simulink model "DC_motor_comparison_28_01"  (R2019a)
settings: Solver=VariableStepAuto  StartTime=0.0  StopTime=50  RelTol=1e-3
undefined symbols (not defined in the file or in its folder): sigbuilder_block
libraries: simulink x4
settings Model: Creator=hp  LastModifiedBy=hp
settings SolverCC: AlgebraicLoopSolver=LineSearch

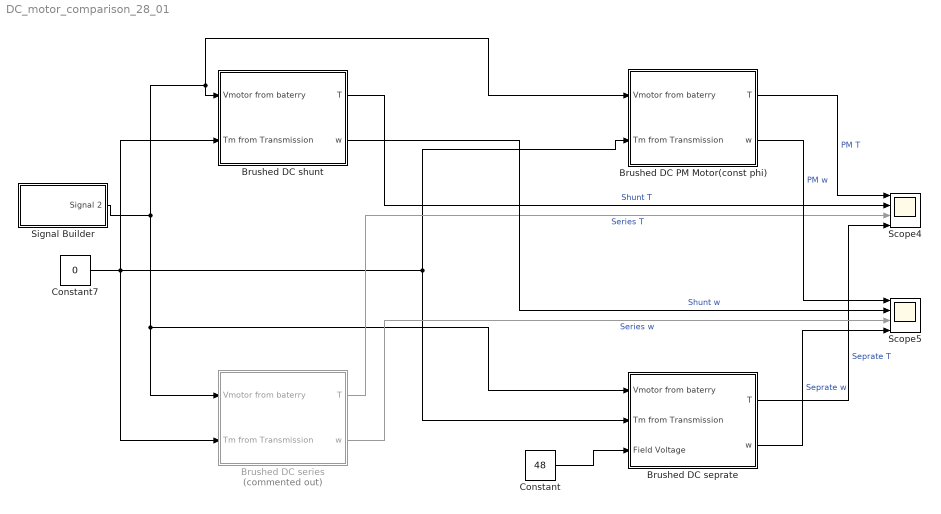
== system DC_motor_comparison_28_01 ==
  Brushed DC PM Motor(const phi) : Subsystem
  Brushed DC seprate : Subsystem
  Brushed DC series : Subsystem  Commented=on
  Brushed DC shunt : Subsystem
  Constant : Constant  Value=48
  Constant7 : Constant  Value=0
  Scope4 : Scope  NumInputPorts=4
  Scope5 : Scope  NumInputPorts=4
  Signal Builder : Subsystem  Tag=STV Subsys  LoadFcn=sigbuilder_block('load',[123.75 80.25 550.5 359.25 ]);  StartFcn=sigbuilder_block('start');  StopFcn=sigbuilder_block('stop');  ClipboardFcn=sigbuilder_block('clipboard');  mask(Sigbuilder block){tuvar=[0:10]}
      mask help: Simulink:masks:SigbuilderBlock_MD
      mask init:
      | if ~strcmp(get_param(bdroot(gcbh),'SimulationStatus'),'stopped') tuvar = sigbuilder_block('maskInit'); end
      settings: CopyFcn=sigbuilder_block('copy');  DeleteFcn=sigbuilder_block('delete');  ModelCloseFcn=sigbuilder_block('modelClose');  PreSaveFcn=sigbuilder_block('preSave');  PauseFcn=sigbuilder_block('pause');  ContinueFcn=sigbuilder_block('continue');  NameChangeFcn=sigbuilder_block('namechange');  OpenFcn=sigbuilder_block('open',[123.75 80.25 550.5 359.25 ]);  CloseFcn=sigbuilder_block('close');
      mask Display: plot(0, 0, 100, 100,[2, 2, 32, 32, 2], [68, 8, 8, 68, 68],[32, 2], [38, 38], [32, 19, 2],[53, 60, 44], [32, 17, 17, 2],[16, 16, 31, 31]);txt = getActiveGroup(gcbh);text(2, 100, txt,'verticalAlignment', 'top');
  wires:
  Signal Builder/1(Signal 2) -> Brushed DC series/1(Vmotor from baterry), Brushed DC seprate/1(Vmotor from baterry), Brushed DC PM Motor(const phi)/1(Vmotor from baterry), Brushed DC shunt/1(Vmotor from baterry)
  Constant7/1 -> Brushed DC series/2(Tm from Transmission), Brushed DC shunt/2(Tm from Transmission), Brushed DC seprate/2(Tm from Transmission), Brushed DC PM Motor(const phi)/2(Tm from Transmission)
  Brushed DC PM Motor(const phi)/1(T) -> Scope4/1  "PM T"
  Brushed DC shunt/1(T) -> Scope4/2  "Shunt T"
  Brushed DC series/1(T) -> Scope4/3  "Series T"
  Brushed DC seprate/1(T) -> Scope4/4  "Seprate T"
  Brushed DC seprate/2(w) -> Scope5/4  "Seprate w"
  Brushed DC series/2(w) -> Scope5/3  "Series w"
  Brushed DC PM Motor(const phi)/2(w) -> Scope5/1  "PM w"
  Brushed DC shunt/2(w) -> Scope5/2  "Shunt w"
  Constant/1 -> Brushed DC seprate/3(Field Voltage)

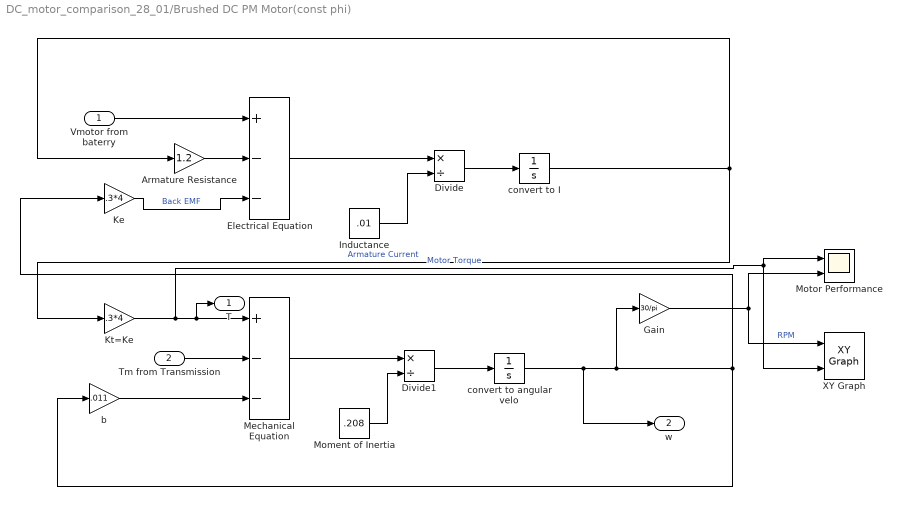
== system DC_motor_comparison_28_01/Brushed DC PM Motor(const phi) ==
  Vmotor from baterry : Inport
  Tm from Transmission : Inport  Port=2
  Armature Resistance : Gain  Gain=1.2
  Divide : Product  Inputs=*/
  Divide1 : Product  Inputs=*/
  Electrical Equation : Sum  Inputs=+--
  Gain : Gain  Gain=30/pi
  Inductance : Constant  Value=.01
  Ke : Gain  Gain=.3*4
  Kt=Ke : Gain  Gain=.3*4
  Mechanical Equation : Sum  Inputs=+--
  Moment of Inertia : Constant  Value=.208
  Motor Performance : Scope  NumInputPorts=2
  XY Graph : simulink/Sinks/XY Graph  xmin=0  xmax=12000  ymin=0  ymax=265  st=-1
  b : Gain  Gain=.011
  convert to angular velo : Integrator
  "convert to I " : Integrator
  T : Outport
  w : Outport  Port=2
  wires:
  Ke/1 -> Electrical Equation/3  "Back EMF"
  Divide/1 -> "convert to I "/1
  Armature Resistance/1 -> Electrical Equation/2
  Electrical Equation/1 -> Divide/1
  Inductance/1 -> Divide/2
  Mechanical Equation/1 -> Divide1/1
  "convert to I "/1 -> Armature Resistance/1, Kt=Ke/1  "Armature Current"
  Kt=Ke/1 -> XY Graph/2, Motor Performance/1, T/1, Mechanical Equation/1  "Motor Torque"
  convert to angular velo/1 -> Ke/1, b/1, Gain/1, w/1
  b/1 -> Mechanical Equation/3
  Moment of Inertia/1 -> Divide1/2
  Tm from Transmission/1 -> Mechanical Equation/2
  Divide1/1 -> convert to angular velo/1
  Vmotor from baterry/1 -> Electrical Equation/1
  Gain/1 -> XY Graph/1, Motor Performance/2  "RPM"

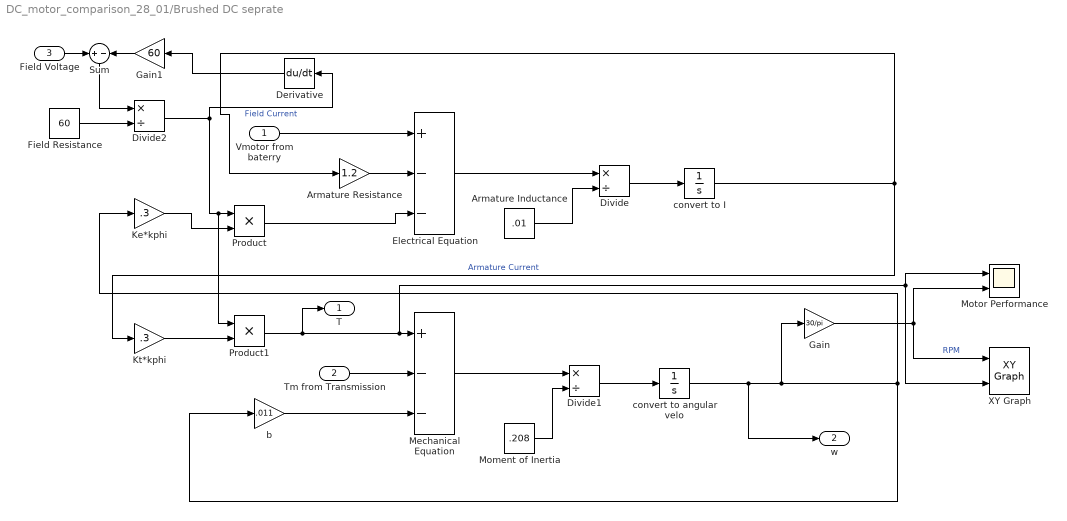
== system DC_motor_comparison_28_01/Brushed DC seprate ==
  Vmotor from baterry : Inport
  Tm from Transmission : Inport  Port=2
  Field Voltage : Inport  Port=3
  Armature Inductance : Constant  Value=.01
  Armature Resistance : Gain  Gain=1.2
  Derivative : Derivative
  Divide : Product  Inputs=*/
  Divide1 : Product  Inputs=*/
  Divide2 : Product  Inputs=*/
  Electrical Equation : Sum  Inputs=+--
  Field Resistance : Constant  Value=60
  Gain : Gain  Gain=30/pi
  Gain1 : Gain  Gain=60
  Ke*kphi : Gain  Gain=.3
  Kt*kphi : Gain  Gain=.3
  Mechanical Equation : Sum  Inputs=+--
  Moment of Inertia : Constant  Value=.208
  Motor Performance : Scope  NumInputPorts=2
  Product : Product
  Product1 : Product
  Sum : Sum  Inputs=+-
  XY Graph : simulink/Sinks/XY Graph  xmin=0  xmax=8000  ymin=0  ymax=25  st=-1
  b : Gain  Gain=.011
  convert to angular velo : Integrator
  "convert to I " : Integrator
  T : Outport
  w : Outport  Port=2
  wires:
  Product1/1 -> T/1, Mechanical Equation/1, Motor Performance/1, XY Graph/2
  Kt*kphi/1 -> Product1/2
  Divide2/1 -> Derivative/1, Product/1, Product1/1  "Field Current"
  Ke*kphi/1 -> Product/2
  Product/1 -> Electrical Equation/3
  Field Resistance/1 -> Divide2/2
  Divide/1 -> "convert to I "/1
  Armature Resistance/1 -> Electrical Equation/2
  Electrical Equation/1 -> Divide/1
  Armature Inductance/1 -> Divide/2
  Mechanical Equation/1 -> Divide1/1
  "convert to I "/1 -> Armature Resistance/1, Kt*kphi/1  "Armature Current"
  convert to angular velo/1 -> Ke*kphi/1, b/1, Gain/1, w/1
  b/1 -> Mechanical Equation/3
  Moment of Inertia/1 -> Divide1/2
  Tm from Transmission/1 -> Mechanical Equation/2
  Divide1/1 -> convert to angular velo/1
  Vmotor from baterry/1 -> Electrical Equation/1
  Gain/1 -> XY Graph/1, Motor Performance/2  "RPM"
  Derivative/1 -> Gain1/1
  Gain1/1 -> Sum/2
  Field Voltage/1 -> Sum/1
  Sum/1 -> Divide2/1

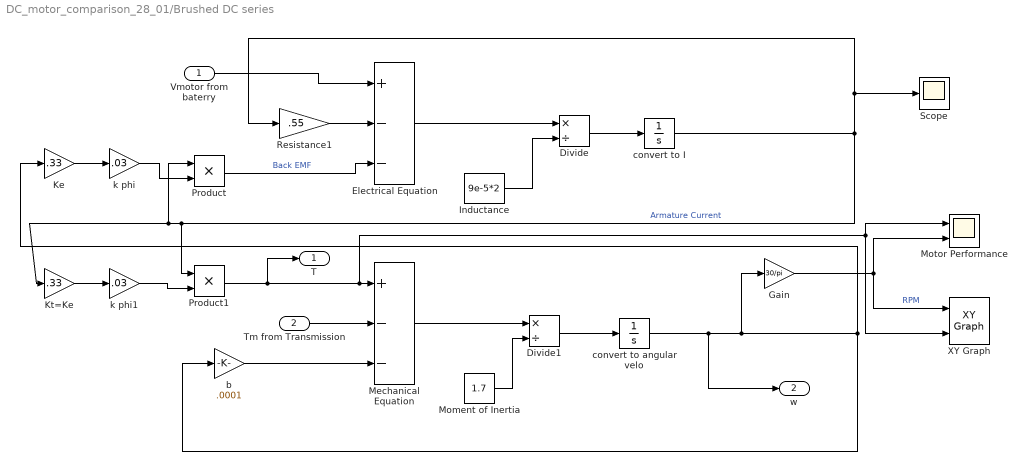
== system DC_motor_comparison_28_01/Brushed DC series ==
  Vmotor from baterry : Inport
  Tm from Transmission : Inport  Port=2
  Divide : Product  Inputs=*/
  Divide1 : Product  Inputs=*/
  Electrical Equation : Sum  Inputs=+--
  Gain : Gain  Gain=30/pi
  Inductance : Constant  Value=9e-5*2
  Ke : Gain  Gain=.33
  Kt=Ke : Gain  Gain=.33
  Mechanical Equation : Sum  Inputs=+--
  Moment of Inertia : Constant  Value=1.7
  Motor Performance : Scope  NumInputPorts=2
  Product : Product
  Product1 : Product
  Resistance1 : Gain  Gain=.55
  Scope : Scope
  XY Graph : simulink/Sinks/XY Graph  xmin=0  xmax=800  ymin=0  ymax=80  st=-1
  b : Gain  Gain=.0001
  convert to angular velo : Integrator
  "convert to I " : Integrator
  k phi : Gain  Gain=.03
  k phi1 : Gain  Gain=.03
  T : Outport
  w : Outport  Port=2
  wires:
  Gain/1 -> Motor Performance/2, XY Graph/1  "RPM"
  Vmotor from baterry/1 -> Electrical Equation/1
  Divide1/1 -> convert to angular velo/1
  Tm from Transmission/1 -> Mechanical Equation/2
  Moment of Inertia/1 -> Divide1/2
  b/1 -> Mechanical Equation/3
  convert to angular velo/1 -> w/1, Gain/1, b/1, Ke/1
  Kt=Ke/1 -> k phi1/1
  "convert to I "/1 -> Product1/1, Product/1, Kt=Ke/1, Resistance1/1, Scope/1  "Armature Current"
  Mechanical Equation/1 -> Divide1/1
  Inductance/1 -> Divide/2
  Electrical Equation/1 -> Divide/1
  Resistance1/1 -> Electrical Equation/2
  Divide/1 -> "convert to I "/1
  Ke/1 -> k phi/1
  k phi/1 -> Product/2
  k phi1/1 -> Product1/2
  Product1/1 -> T/1, XY Graph/2, Motor Performance/1, Mechanical Equation/1
  Product/1 -> Electrical Equation/3  "Back EMF"

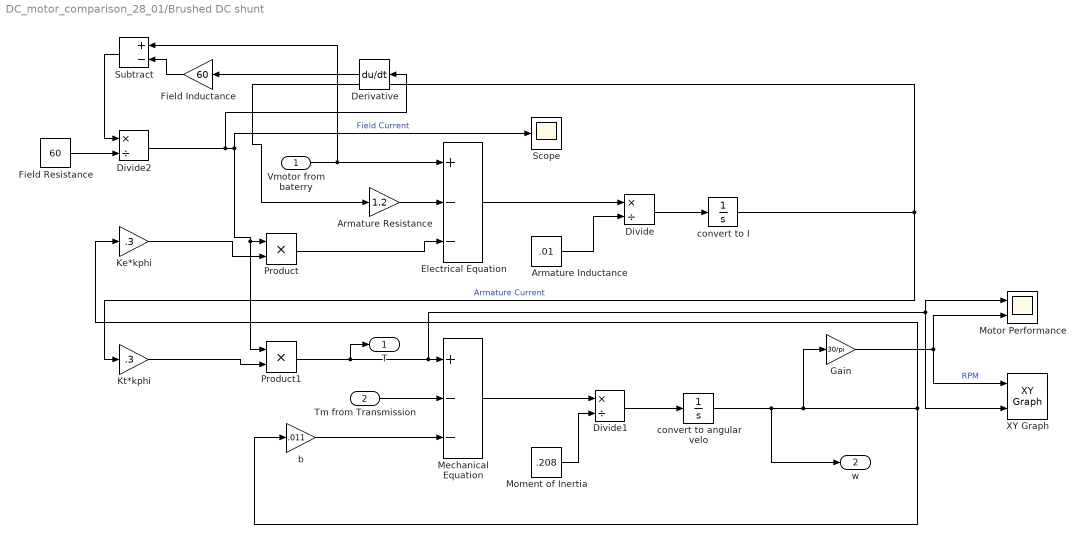
== system DC_motor_comparison_28_01/Brushed DC shunt ==
  Vmotor from baterry : Inport
  Tm from Transmission : Inport  Port=2
  Armature Inductance : Constant  Value=.01
  Armature Resistance : Gain  Gain=1.2
  Derivative : Derivative
  Divide : Product  Inputs=*/
  Divide1 : Product  Inputs=*/
  Divide2 : Product  Inputs=*/
  Electrical Equation : Sum  Inputs=+--
  Field Inductance : Gain  Gain=60
  Field Resistance : Constant  Value=60
  Gain : Gain  Gain=30/pi
  Ke*kphi : Gain  Gain=.3
  Kt*kphi : Gain  Gain=.3
  Mechanical Equation : Sum  Inputs=+--
  Moment of Inertia : Constant  Value=.208
  Motor Performance : Scope  NumInputPorts=2
  Product : Product
  Product1 : Product
  Scope : Scope
  Subtract : Sum  Inputs=+-
  XY Graph : simulink/Sinks/XY Graph  xmin=0  xmax=800  ymin=0  ymax=80  st=-1
  b : Gain  Gain=.011
  convert to angular velo : Integrator
  "convert to I " : Integrator
  T : Outport
  w : Outport  Port=2
  wires:
  Product1/1 -> T/1, Mechanical Equation/1, Motor Performance/1, XY Graph/2
  Kt*kphi/1 -> Product1/2
  Divide2/1 -> Derivative/1, Scope/1, Product/1, Product1/1  "Field Current"
  Ke*kphi/1 -> Product/2
  Product/1 -> Electrical Equation/3
  Field Resistance/1 -> Divide2/2
  Divide/1 -> "convert to I "/1
  Armature Resistance/1 -> Electrical Equation/2
  Electrical Equation/1 -> Divide/1
  Armature Inductance/1 -> Divide/2
  Mechanical Equation/1 -> Divide1/1
  "convert to I "/1 -> Armature Resistance/1, Kt*kphi/1  "Armature Current"
  convert to angular velo/1 -> Ke*kphi/1, b/1, Gain/1, w/1
  b/1 -> Mechanical Equation/3
  Moment of Inertia/1 -> Divide1/2
  Tm from Transmission/1 -> Mechanical Equation/2
  Divide1/1 -> convert to angular velo/1
  Vmotor from baterry/1 -> Subtract/1, Electrical Equation/1
  Gain/1 -> XY Graph/1, Motor Performance/2  "RPM"
  Field Inductance/1 -> Subtract/2
  Derivative/1 -> Field Inductance/1
  Subtract/1 -> Divide2/1

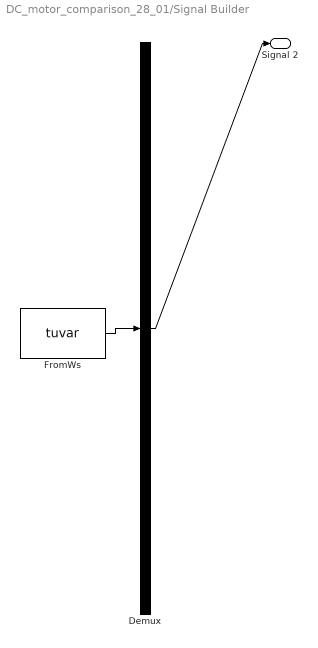
== system DC_motor_comparison_28_01/Signal Builder ==
  Demux : Demux  Tag=STV Demux  Outputs=1
  FromWs : FromWorkspace  Tag=STV FromWs  VariableName=tuvar  SampleTime=0
      SigBuilderData=|
      | common.afterFinalStr = 'Extrapolate'
      | common.sampleTime = 0
      | dataSet.timeRange = [0 50]
      | dataSet.name = 'Group 1'
      | sbobj.Groups.Name = 'Group 1'
      | sbobj.Groups.Signals.Name = 'Signal 2'
      | sbobj.Groups.Signals.XData = [0 10 50]
      | sbobj.Groups.Signals.YData = [0 240 240]
      | sbobj.Groups.TimeRange = [0 50]
  Signal 2 : Outport  Tag=STV Outport
  wires:
  FromWs/1 -> Demux/1
  Demux/1 -> Signal 2/1
